simulink model "q4"  (R2020b)
settings: Solver=FixedStepAuto  StartTime=0.0  StopTime=5.0  FixedStep=.0002  RelTol=1e-3
settings Model: Creator=Frienddo  LastModifiedBy=Frienddo

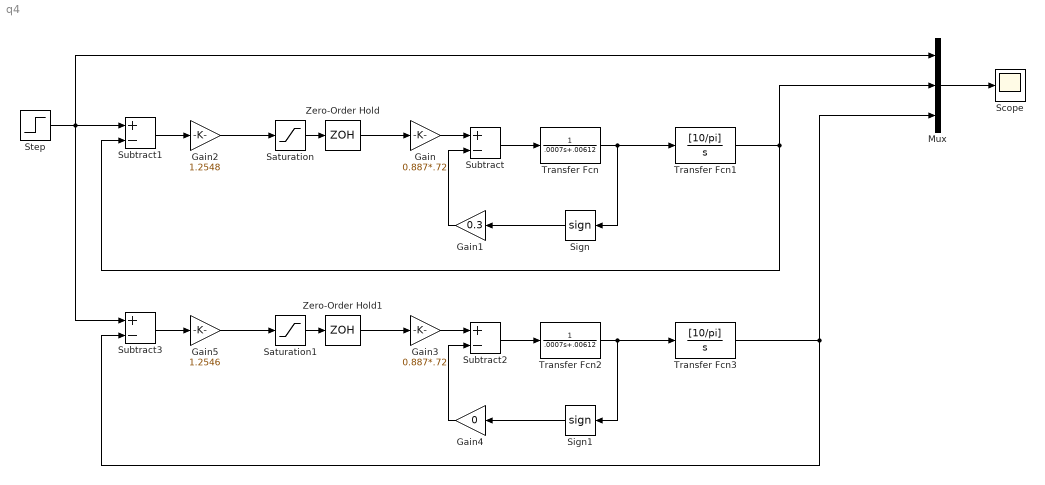
== system q4 ==
  Gain : Gain  Gain=0.887*.72
  Gain1 : Gain  Gain=0.3
  Gain2 : Gain  Gain=1.2548
  Gain3 : Gain  Gain=0.887*.72
  Gain4 : Gain  Gain=0
  Gain5 : Gain  Gain=1.2546
  Mux : Mux  Inputs=3
  Saturation : Saturate  UpperLimit=3  LowerLimit=-3
  Saturation1 : Saturate  UpperLimit=3  LowerLimit=-3
  Scope : Scope
  Sign : Signum
  Sign1 : Signum
  Step : Step  SampleTime=0
  Subtract{,1..3} (4 alike) : Sum  Inputs=+-
  Transfer Fcn : TransferFcn  Denominator=[.0007 .00612]
  Transfer Fcn1 : TransferFcn  Numerator=[10/pi]  Denominator=[1 0]
  Transfer Fcn2 : TransferFcn  Denominator=[.0007 .00612]
  Transfer Fcn3 : TransferFcn  Numerator=[10/pi]  Denominator=[1 0]
  Zero-Order Hold : ZeroOrderHold  SampleTime=.0002
  Zero-Order Hold1 : ZeroOrderHold  SampleTime=.0002
  wires:
  Saturation/1 -> Zero-Order Hold/1
  Gain/1 -> Subtract/1
  Subtract/1 -> Transfer Fcn/1
  Transfer Fcn/1 -> Sign/1, Transfer Fcn1/1
  Sign/1 -> Gain1/1
  Gain1/1 -> Subtract/2
  Gain2/1 -> Saturation/1
  Zero-Order Hold/1 -> Gain/1
  Transfer Fcn1/1 -> Subtract1/2, Mux/2
  Subtract1/1 -> Gain2/1
  Mux/1 -> Scope/1
  Step/1 -> Subtract3/1, Mux/1, Subtract1/1
  Transfer Fcn3/1 -> Mux/3, Subtract3/2
  Subtract3/1 -> Gain5/1
  Sign1/1 -> Gain4/1
  Zero-Order Hold1/1 -> Gain3/1
  Gain4/1 -> Subtract2/2
  Transfer Fcn2/1 -> Sign1/1, Transfer Fcn3/1
  Gain3/1 -> Subtract2/1
  Gain5/1 -> Saturation1/1
  Saturation1/1 -> Zero-Order Hold1/1
  Subtract2/1 -> Transfer Fcn2/1
